simulink model "dvfs_zed_simple"  (R2025b)
settings: Solver=FixedStepDiscrete  StartTime=0.0  StopTime=10.0  FixedStep=0.1  RelTol=1e-3
model workspace (MAT data in the model file):
  workload_vec = 1
settings Model: Creator=Vimal Rency  LastModifiedBy=Vimal Rency
settings OptimizationCC: BlockReduction=off  ConditionallyExecuteInputs=off  DefaultParameterBehavior=Inlined
settings HardwareCC: ProdBitPerPointer=32.0  ProdBitPerSizeT=32.0  ProdBitPerPtrDiffT=32.0  ProdLargestAtomicFloat=None  ProdIntDivRoundTo=Undefined  ProdEndianess=Unspecified  ProdWordSize=32.0  ProdHWDeviceType=ASIC/FPGA->ASIC/FPGA  TargetBitPerPointer=64.0  TargetBitPerSizeT=64.0  TargetBitPerPtrDiffT=64.0  TargetLongLongMode=on  TargetIntDivRoundTo=Zero  TargetEndianess=LittleEndian  TargetWordSize=64.0  TargetHWDeviceType=Custom Processor->MATLAB Host Computer  ProdEqTarget=off

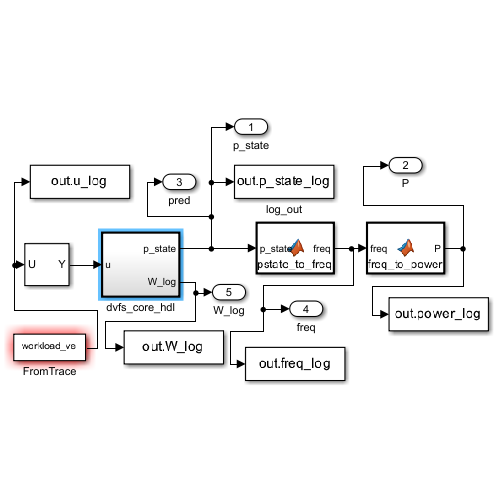
[thumbnail: Simulink's stored preview of the top-level diagram]
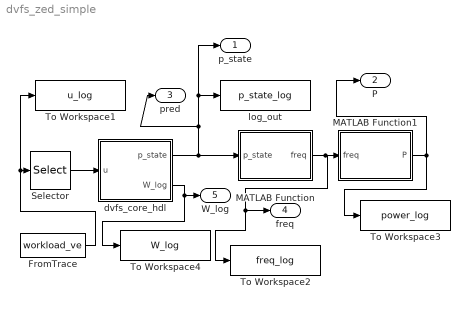
== system dvfs_zed_simple ==
  FromTrace : FromWorkspace  VariableName=workload_ve
  MATLAB Function : MATLAB Function  TreatAsAtomicUnit=on
  MATLAB Function1 : MATLAB Function  TreatAsAtomicUnit=on
  Selector : Selector  NumberOfDimensions=2  InputPortWidth=3  IndexOptions=Select all,Index vector (dialog)  Indices=[1 3],1  OutputSizes=1,1
  To Workspace1 : ToWorkspace  VariableName=u_log  SampleTime=-1
  To Workspace2 : ToWorkspace  VariableName=freq_log  SampleTime=-1
  To Workspace3 : ToWorkspace  VariableName=power_log  SampleTime=-1
  To Workspace4 : ToWorkspace  VariableName=W_log  SampleTime=-1
  dvfs_core_hdl : Subsystem  TreatAsAtomicUnit=on  SystemSampleTime=0.1
  log_out : ToWorkspace  VariableName=p_state_log  SampleTime=-1
  p_state : Outport
  P : Outport  Port=2
  pred : Outport  Port=3
  freq : Outport  Port=4
  W_log : Outport  Port=5
  wires:
  FromTrace/1 -> To Workspace1/1, Selector/1
  MATLAB Function1/1(P) -> To Workspace3/1, P/1
  MATLAB Function/1(freq) -> To Workspace2/1, freq/1, MATLAB Function1/1(freq)
  dvfs_core_hdl/2(W_log) -> To Workspace4/1, W_log/1
  dvfs_core_hdl/1(p_state) -> p_state/1, log_out/1, pred/1, MATLAB Function/1(p_state)
  Selector/1 -> dvfs_core_hdl/1(u)

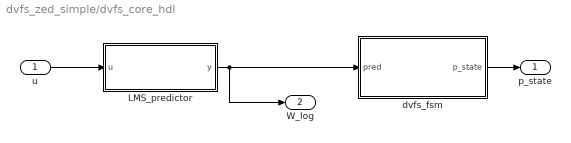
== system dvfs_zed_simple/dvfs_core_hdl ==
  u : Inport
  LMS_predictor : MATLAB Function  TreatAsAtomicUnit=on  SystemSampleTime=0.1
  dvfs_fsm : MATLAB Function  TreatAsAtomicUnit=on
  p_state : Outport
  W_log : Outport  Port=2
  wires:
  dvfs_fsm/1(p_state) -> p_state/1
  LMS_predictor/1(y) -> W_log/1, dvfs_fsm/1(pred)
  u/1 -> LMS_predictor/1(u)

== matlab function dvfs_zed_simple/dvfs_core_hdl/LMS_predictor ==
  data: u input; y output
function y = LMS_predictor(u)
%#codegen

% Cast input to single to avoid type mismatch
u = single(u);

persistent prev
if isempty(prev)
    prev = single(0); 
end

W = single(0.8);     % fixed weight
bias = single(0.02); % fixed bias

% Prediction
y = W * prev + bias;

% Update state
prev = u;

% Clamp result
if y < 0
    y = single(0);
elseif y > 1
    y = single(1);
end

== matlab function dvfs_zed_simple/MATLAB Function ==
  data: p_state input; freq output
function freq = pstate_to_freq(p_state)

switch p_state
    case 0
        freq = 100;   % MHz
    case 1
        freq = 200;
    case 2
        freq = 300;
    otherwise
        freq = 0;
end

end

== matlab function dvfs_zed_simple/MATLAB Function1 ==
  data: freq input; P output
function P = freq_to_power(freq)

% simple model: Power ∝ frequency
P = 0.01 * freq;   % scale as you want (mW)

end

== matlab function dvfs_zed_simple/dvfs_core_hdl/dvfs_fsm ==
  data: pred input; p_state output
function p_state = dvfs_fsm(pred)
% 0=LOW, 1=MED, 2=HIGH

persistent state last_change cycle_cnt next_avail
if isempty(state)
    state = uint8(1); % start in MED
    last_change = uint32(0);
    cycle_cnt = uint32(0);
    next_avail = uint32(0);
end

cycle_cnt = cycle_cnt + 1;

T1 = 0.08;
T2 = 0.26;
H  = 0.02;
min_residency = uint32(0);
transition_latency = uint32(0);

desired = state;

switch state
    case uint8(0)        % LOW
        if pred >= T1 + H
            desired = uint8(1);
        end
    case uint8(1)        % MED
        if pred >= T2 + H
            desired = uint8(2);
        elseif pred < T1 - H
            desired = uint8(0);
        end
    case uint8(2)        % HIGH
        if pred < T2 - H
            desired = uint8(1);
        end
end

if desired ~= state
    state = desired;
    last_change = cycle_cnt;
    next_avail = cycle_cnt;
end


p_state = state;
end
